simulink model "ECE411_prj_OpenCircuitRotorSpinUp"  (R2023b)
settings: Solver=VariableStepAuto  StartTime=0.0  StopTime=2  RelTol=1e-3
values from neighbouring files (symbols this model uses):
  P = 8    [ECE411_HW2_2_Parameters.m]    (also in main_code.m)
  RPM_max = 4259    [ECE411_HW2_2_Parameters.m]    (also in ECE411_Project_Parameters_Starter.m = 3700; main_code.m = 3700)
libraries: fl_lib x9, nesl_utility x7, ee_lib x1, simulink x1
settings Model: SimulationMode=accelerator  Creator=DiggerPC  LastModifiedBy=baik3-ad
settings DebuggingCC: UnconnectedInputMsg=warning  UnconnectedOutputMsg=warning  UnconnectedLineMsg=warning
settings ModelReferenceCC: EnableRefExpFcnMdlSchedulingChecks=on
settings RTWCC: DLArmComputeVersion=19.05

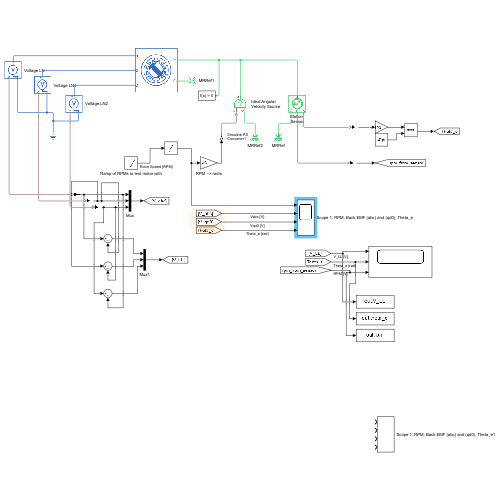
[thumbnail: Simulink's stored preview of the top-level diagram]
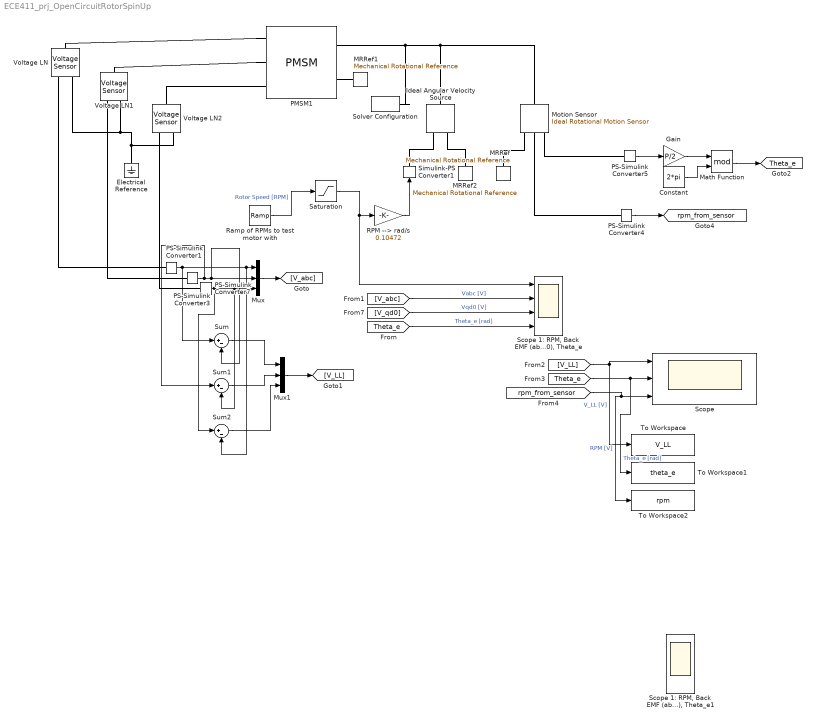
== system ECE411_prj_OpenCircuitRotorSpinUp ==
  Constant : Constant  Value=2*pi
  Electrical Reference : fl_lib/Electrical/Electrical Elements/Electrical Reference
  Gain : Gain  Gain=P/2
  Ideal Angular Velocity Source : fl_lib/Mechanical/Mechanical Sources/Ideal Angular Velocity Source
  MRRef : fl_lib/Mechanical/Rotational Elements/Mechanical Rotational Reference
  MRRef1 : fl_lib/Mechanical/Rotational Elements/Mechanical Rotational Reference
  MRRef2 : fl_lib/Mechanical/Rotational Elements/Mechanical Rotational Reference
  Math Function : Math  Operator=mod
  Motion Sensor : fl_lib/Mechanical/Mechanical Sensors/Ideal Rotational Motion Sensor  reference=foundation.enum.MeasurementReference.difference  acceleration_port=false  velocity_port=true  position_port=true  wrap_angle=simscape.enum.onoff.on  offset=0 deg
  Mux : Mux  Inputs=3
  Mux1 : Mux  Inputs=3
  PMSM1 : ee_lib/Electromechanical/Permanent Magnet/PMSM  port_option=ee.enum.threePhasePort.expanded  winding_type=ee.enum.statorconnection.wye  machine_param=ee.enum.pmsm.parameterization.constant  nPolePairs=P/2  pmflux_param=ee.enum.pmflux.fluxlinkage  pm_flux_linkage=lambda_f Wb  torque_constant=0.037*sqrt(2) N*m/A  back_emf_constant=0.037*sqrt(2) V/(rad/s)  stator_param=ee.enum.statorparam.LdLqL0  Ld=Lq H  Lq=Ld H  idVec=[-200, 0, 200] A  iqVec=[-200, 0, 200] A  LdMatrix=0.0002 * ones(3, 3) H  LqMatrix=0.0002 * ones(3, 3) H  PmMatrix=0.1 * ones(3, 3) Wb  ktMatrix=0.18 * ones(3, 3) N*m/A  keMatrix=0.18 * ones(3, 3) V/(rad/s)  L0=L0 H  Ls=Ls H  Lm=0 H  Ms=0 H  Rs=Rs Ohm  zero_sequence=ee.enum.park.zerosequence.exclude  axes_param=ee.enum.rotorangle.qaxis  loss_param=ee.enum.ironloss.none  losses_oc=[0, 0, 0] W  losses_sc=[0, 0, 0] W  f_losses=60 Hz  Isc_losses=95 A  J=0.01 kg*m^2  lam=0 N*m/(rad/s)  i_d_specify=off  i_d_priority=None  i_d=0 A  i_d_nominal_specify=off  i_d_nominal_unit=A  i_d_nominal_value=1  i_q_specify=off  i_q_priority=None  i_q=0 A  i_q_nominal_specify=off  i_q_nominal_unit=A  i_q_nominal_value=1  torque_specify=off  torque_priority=None  torque=0 N*m  torque_nominal_specify=off  torque_nominal_unit=N*m  torque_nominal_value=1  angular_velocity_specify=off  angular_velocity_priority=High  angular_velocity=0 rpm  angular_velocity_nominal_specify=off  angular_velocity_nominal_unit=rpm  angular_velocity_nominal_value=1  angular_position_specify=off  angular_position_priority=High  angular_position=0 deg  angular_position_nominal_specify=off  angular_position_nominal_unit=deg  angular_position_nominal_value=1  alpha=3.93e-3 1/K  alpha_flux=-0.001 1/K  Tmeas=298.15 K  stator_thermal_mass=100 J/K  rotor_thermal_mass=200 J/K  Rm_percent_rotor=90  Rd_percent_rotor=30  temperatureA_specify=off  temperatureA_priority=High  temperatureA=25 degC  temperatureA_nominal_specify=off  temperatureA_nominal_unit=degC  temperatureA_nominal_value=1  temperatureB_specify=off  temperatureB_priority=High  temperatureB=25 degC  temperatureB_nominal_specify=off  temperatureB_nominal_unit=degC  temperatureB_nominal_value=1  temperatureC_specify=off  temperatureC_priority=High  temperatureC=25 degC  temperatureC_nominal_specify=off  temperatureC_nominal_unit=degC  temperatureC_nominal_value=1  temperatureR_specify=off  temperatureR_priority=High  temperatureR=25 degC  temperatureR_nominal_specify=off  temperatureR_nominal_unit=degC  temperatureR_nominal_value=1
      settings: InternalSimscapePortConfiguration="{\"Bottom\":[],\"Left\":[{\"id\":\"a\",\"label\":\"a\",\"type\":\"foundation.electrical.electrical\"},{\"id\":\"b\",\"label\":\"b\",\"type\":\"foundation.electrical.electrical\"},{\"id\":\"c\",\"label\":\"c\",\"type\":\"foundation.electrical.electrical\"}],\"Right\":[{\"id\":\"R\",\"label\":\"R\",\"type\":\"foundation.mechanical.rotational.rotational\"},{\"id\":\"C\",\"label\":\"C\",\"type\":\"foundation.mechanical.rotational.rotational\"}],\"Top\":[]}"
  PS-Simulink Converter1 : nesl_utility/PS-Simulink Converter  PhysicalDomain=network_engine_domain  SubClassName=ps_output  LeftPortType=input  RightPortType=output  PseudoPeriodic=off  Frequencies=[]  VectorFormat=1-D array  Unit=V  AffineConversion=off
  PS-Simulink Converter3 : nesl_utility/PS-Simulink Converter  PhysicalDomain=network_engine_domain  SubClassName=ps_output  LeftPortType=input  RightPortType=output  PseudoPeriodic=off  Frequencies=[]  VectorFormat=1-D array  Unit=V  AffineConversion=off
  PS-Simulink Converter4 : nesl_utility/PS-Simulink Converter  PhysicalDomain=network_engine_domain  SubClassName=ps_output  LeftPortType=input  RightPortType=output  PseudoPeriodic=off  Frequencies=[]  VectorFormat=1-D array  Unit=rpm  AffineConversion=off
  PS-Simulink Converter5 : nesl_utility/PS-Simulink Converter  PhysicalDomain=network_engine_domain  SubClassName=ps_output  LeftPortType=input  RightPortType=output  PseudoPeriodic=off  Frequencies=[]  VectorFormat=1-D array  Unit=rad  AffineConversion=off
  PS-Simulink Converter7 : nesl_utility/PS-Simulink Converter  PhysicalDomain=network_engine_domain  SubClassName=ps_output  LeftPortType=input  RightPortType=output  PseudoPeriodic=off  Frequencies=[]  VectorFormat=1-D array  Unit=V  AffineConversion=off
  RPM --> rad/s : Gain  Gain=0.10472
  Ramp of RPMs to test motor with : simulink/Sources/Ramp  slope=RPM_max  start=0  InitialOutput=0
  Saturation : Saturate  UpperLimit=4259  LowerLimit=0
  Scope : Scope  NumInputPorts=3
  "Scope 1: RPM, Back EMF (abc) and (qd0), Theta_e" : Scope  NumInputPorts=4
  "Scope 1: RPM, Back EMF (abc) and (qd0), Theta_e1" : Scope  NumInputPorts=4
  Simulink-PS Converter1 : nesl_utility/Simulink-PS Converter  PhysicalDomain=network_engine_domain  SubClassName=ps_input  LeftPortType=input  RightPortType=output  PseudoPeriodic=off  Frequencies=[]  NoiseDistribution=none  NoiseParameters=[]  Unit=rad/s  AffineConversion=off  FilteringAndDerivatives=zero  SimscapeFilterOrder=1  InputFilterTimeConstant=0.001  UdotUserProvided=1
  Solver Configuration : nesl_utility/Solver Configuration  PhysicalDomain=network_engine_domain  SubClassName=solver  LeftPortType=input  RightPortType=generic  Tones=[]  Harmonics=[]  SimulateNoise=off  Profile=off  UseLocalSampling=off  EnableSwitchedLinearOptims=on  FrequencyDomain=off  UseCCode=off  RelTol=0.001  AbsTol=1e-06  MinStep=1e-09  ToWorkspace=off  RevertToSquareIcSolve=off  NumHomotopyIterations=100  PhasorMode=off  PhasorModeNumHarmonics=1  ConsistencySolver=NEWTON_FTOL  IndexReductionMethod=DerivativeReplacement  DoDC=off  ResidualTolerance=1e-09  ConsistencyTolSource=GLOBAL  ConsistencyAbsTol=0.001  ConsistencyRelTol=0.001  ConsistencyTolFactor=0.001  UseLocalSolver=on  LocalSolverChoice=NE_TRAPEZOIDAL_ADVANCER  ResolveIndetEquations=on  FunctionEvalNumThread=1  LocalSolverSampleTime=1e-6  DoFixedCost=on  MaxNonlinIter=3  MaxModeIter=2  ComputeImpulses=off  ImpulseIterations=2  LinearAlgebra=auto  LinearAlgebraNumThread=0  EquationFormulation=NE_TIME_EF  DelaysMemoryBudget=1024  AutomaticFiltering=on  FilteringTimeConstant=0.001  PartitionStorageMethod=AS_NEEDED  PartitionMemoryBudget=1024  PartitionMethod=ROBUST  MultibodyUseLocalSolver=off  MultibodyLocalSolverChoice=ODE1  MultibodyLocalSolverSampleTime=0.001
  Sum : Sum  Inputs=|+-
  Sum1 : Sum  Inputs=|+-
  Sum2 : Sum  Inputs=|+-
  To Workspace : ToWorkspace  VariableName=V_LL  SaveFormat=Timeseries  SampleTime=-1
      settings: Save2DSignal=2-D array (concatenate along first dimension)
  To Workspace1 : ToWorkspace  VariableName=theta_e  SaveFormat=Timeseries  SampleTime=-1
      settings: Save2DSignal=2-D array (concatenate along first dimension)
  To Workspace2 : ToWorkspace  VariableName=rpm  SaveFormat=Timeseries  SampleTime=-1
  Voltage LN : fl_lib/Electrical/Electrical Sensors/Voltage Sensor
  Voltage LN1 : fl_lib/Electrical/Electrical Sensors/Voltage Sensor
  Voltage LN2 : fl_lib/Electrical/Electrical Sensors/Voltage Sensor
  tag scope: Theta_e=global, rpm_from_sensor=global
  wires:
  Mux/1 -> [V_abc]
  RPM --> rad/s/1 -> Simulink-PS Converter1/1
  PS-Simulink Converter4/1 -> [rpm_from_sensor]
  PS-Simulink Converter3/1 -> Sum1/1, Sum/2, Mux/2
  PS-Simulink Converter1/1 -> Sum2/2, Mux/1, Sum/1
  Ramp of RPMs to test motor with/1 -> Saturation/1  "Rotor Speed [RPM]"
  PS-Simulink Converter5/1 -> Gain/1
  PS-Simulink Converter7/1 -> Sum2/1, Sum1/2, Mux/3
  [V_qd0] -> "Scope 1: RPM, Back EMF (abc) and (qd0), Theta_e"/3  "Vqd0 [V]"
  Gain/1 -> Math Function/1
  [V_abc] -> "Scope 1: RPM, Back EMF (abc) and (qd0), Theta_e"/2  "Vabc [V]"
  [Theta_e] -> "Scope 1: RPM, Back EMF (abc) and (qd0), Theta_e"/4  "Theta_e [rad]"
  Math Function/1 -> [Theta_e]
  Constant/1 -> Math Function/2
  Saturation/1 -> "Scope 1: RPM, Back EMF (abc) and (qd0), Theta_e"/1, RPM --> rad/s/1
  Sum/1 -> Mux1/1
  Sum1/1 -> Mux1/2
  Sum2/1 -> Mux1/3
  Mux1/1 -> [V_LL]
  [V_LL] -> To Workspace/1, Scope/1  "V_LL [V]"
  [Theta_e] -> To Workspace1/1, Scope/2  "Theta_e [rad]"
  [rpm_from_sensor] -> Scope/3, To Workspace2/1  "RPM [V]"
  connections:
  Motion Sensor/LConn1 -- Ideal Angular Velocity Source/LConn1 -- PMSM1/RConn1 -- Solver Configuration/RConn1
  Simulink-PS Converter1/RConn1 -- Ideal Angular Velocity Source/RConn1
  Voltage LN/RConn1 -- PS-Simulink Converter1/LConn1
  Motion Sensor/RConn3 -- PS-Simulink Converter5/LConn1
  MRRef/LConn1 -- Motion Sensor/RConn1
  Motion Sensor/RConn2 -- PS-Simulink Converter4/LConn1
  MRRef2/LConn1 -- Ideal Angular Velocity Source/RConn2
  PMSM1/RConn2 -- MRRef1/LConn1
  PMSM1/LConn1 -- Voltage LN/LConn1
  PMSM1/LConn3 -- Voltage LN2/LConn1
  PMSM1/LConn2 -- Voltage LN1/LConn1
  PS-Simulink Converter3/LConn1 -- Voltage LN1/RConn1
  PS-Simulink Converter7/LConn1 -- Voltage LN2/RConn1
  Voltage LN/RConn2 -- Voltage LN1/RConn2 -- Voltage LN2/RConn2 -- Electrical Reference/LConn1
